simulink model "rlQubeServo"  (R2025a)
settings: Solver=ode23t  StartTime=0.0  StopTime=10.0  RelTol=1e-3  AbsTol=1e-3
values from neighbouring files (symbols this model uses):
  dphi0 = 0    [TrainAgentsToControlQuanserQUBEPendulumExample.m]    (also in training_1.mat)
  dtheta0 = 0    [TrainAgentsToControlQuanserQUBEPendulumExample.m]    (also in training_1.mat)
  dtheta_limit = 30    [TrainAgentsToControlQuanserQUBEPendulumExample.m]    (also in training_1.mat)
  phi0 = pi-pi/4+rand*pi/2    [TrainAgentsToControlQuanserQUBEPendulumExample.m]    (also in training_1.mat = 0)
  theta0 = -pi/4+rand*pi/2    [TrainAgentsToControlQuanserQUBEPendulumExample.m]    (also in training_1.mat = 0)
  theta_limit = 5*pi/8    (= 1.96349540849)    [TrainAgentsToControlQuanserQUBEPendulumExample.m]    (also in training_1.mat)
  Ts = 0.005    [TrainAgentsToControlQuanserQUBEPendulumExample.m]    (also in training_1.mat)
  volt_limit = 12    [TrainAgentsToControlQuanserQUBEPendulumExample.m]    (also in training_1.mat)
libraries: simulink x2, QuanserQube x1, rllib x1
settings Model: Creator=The MathWorks, Inc.  LastModifiedBy=The MathWorks, Inc.
settings SolverCC: AutoScaleAbsTol=off  MaxZcPerStep=1.0
settings DebuggingCC: UnconnectedInputMsg=warning  UnconnectedOutputMsg=warning  UnconnectedLineMsg=warning
settings ModelReferenceCC: EnableRefExpFcnMdlSchedulingChecks=on
settings RTWCC: GPUComputeCapability=3.5  DLArmComputeVersion=19.05
settings ExplorerConfigSet: InternalSimMechanicsExplorerSettings="<ExplorerConfiguration><canonicalview>default</canonicalview><AnimationSetting><BasePlaybackSpeed>1.0</BasePlaybackSpeed><PlaybackSpeedFactor>1.0</PlaybackSpeedFactor></AnimationSetting><TilePanel><TileInfo><Tiles Columns=\"1\" Count=\"1\" Rows=\"1\"><Column Weight=\"1\"/><Row Weight=\"1\"/><Tile Height=\"1\" Width=\"1\" X=\"0\" Y=\"0\"/></Tiles></TileInfo><SceneInfo><SceneViewer><BGColor><R>0.60000002384185791</R><G>0.60000002384185791</G><B>0.60000002384185791</B></BGColor><Camera><DoPerspective>on</DoPerspective><Position><X>0.334156231583514596</X><Y>0.107146061295956732</Y><Z>0.154419804164132285</Z></Position><Center><X>0.145480827141795971</X><Y>0.0537418892551446009</Y><Z>0.077934111254939889</Z></Center><Up><X>-0.332530024195597795</X><Y>-0.157027945704575345</Y><Z>0.929927958110882913</Z></Up><ViewLimDist>1</ViewLimDist><YLim>0.466307658154998583</YLim><XLim>0.535390274177961367</XLim></Camera></SceneViewer></SceneInfo></TilePanel><MechEditorPanel><Cameras><Camera><Id>Camera1</Id><Value><Name>Camera1</Name><NativeCamera><PositionKeyframeSet/><CenterKeyframeSet/><UpVectorKeyframeSet/></NativeCamera></Value></Camera></Cameras><GfxPanelCameraMap><MapElement CameraMLId=\"Camera1\" GfxPanelIndex=\"0\"/></GfxPanelCameraMap><VideoCreator><PlaybackSpeedRatio>1.0</PlaybackSpeedRatio><FrameRate>30</FrameRate><VideoFormat>Motion JPEG AVI</VideoFormat><FrameSize>auto</FrameSize></VideoCreator></MechEditorPanel></ExplorerConfiguration>"

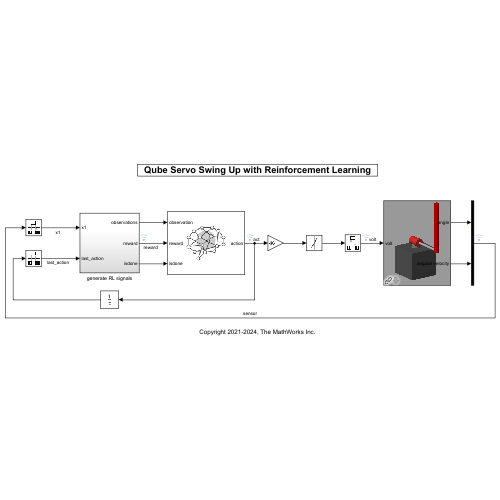
[thumbnail: Simulink's stored preview of the top-level diagram]
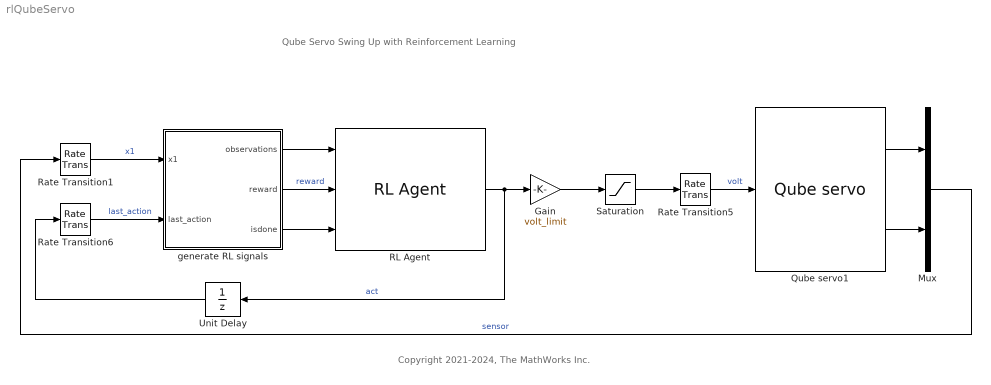
== system rlQubeServo ==
  note: Qube Servo Swing Up with Reinforcement Learning
  note: Copyright 2021-2024, The MathWorks Inc.
  Gain : Gain  Gain=volt_limit
  Mux : Mux  Inputs=2
  Qube servo1 : QuanserQube/Qube servo  a0=[theta0, phi0]  w0=[dtheta0,dphi0]  R_m=8.4  L_m=1.16e-3  mu_m=3e-6  K_b=0.042  n=1  rod_mass=0.095  rod_length=0.103  rod_rad=0.003  p_mass=0.024  p_length=0.129  p_rad=0.0045  D_r=0.001  D_p=5e-6  Choice_Stopper=On
  RL Agent : rllib/RL Agent  Agent=agent  ExternalActionAsInput=off  ProvideLastAction=off  ProvideCumRwd=off  TreatAsDirectFeedthrough=on  UseStrictObservationDataTypes=off
  Rate Transition1 : RateTransition  OutPortSampleTime=Ts
  Rate Transition5 : RateTransition
  Rate Transition6 : RateTransition  OutPortSampleTime=Ts
  Saturation : Saturate  UpperLimit=volt_limit  LowerLimit=-volt_limit
  Unit Delay : UnitDelay  SampleTime=-1  HasFrameUpgradeWarning=on
  generate RL signals : Subsystem
  wires:
  generate RL signals/3(isdone) -> RL Agent/3
  generate RL signals/2(reward) -> RL Agent/2  "reward"
  Qube servo1/1 -> Mux/1
  RL Agent/1 -> Gain/1, Unit Delay/1  "act"
  Qube servo1/2 -> Mux/2
  generate RL signals/1(observations) -> RL Agent/1
  Rate Transition1/1 -> generate RL signals/1(x1)  "x1"
  Unit Delay/1 -> Rate Transition6/1
  Mux/1 -> Rate Transition1/1  "sensor"
  Rate Transition6/1 -> generate RL signals/2(last_action)  "last_action"
  Saturation/1 -> Rate Transition5/1
  Rate Transition5/1 -> Qube servo1/1  "volt"
  Gain/1 -> Saturation/1

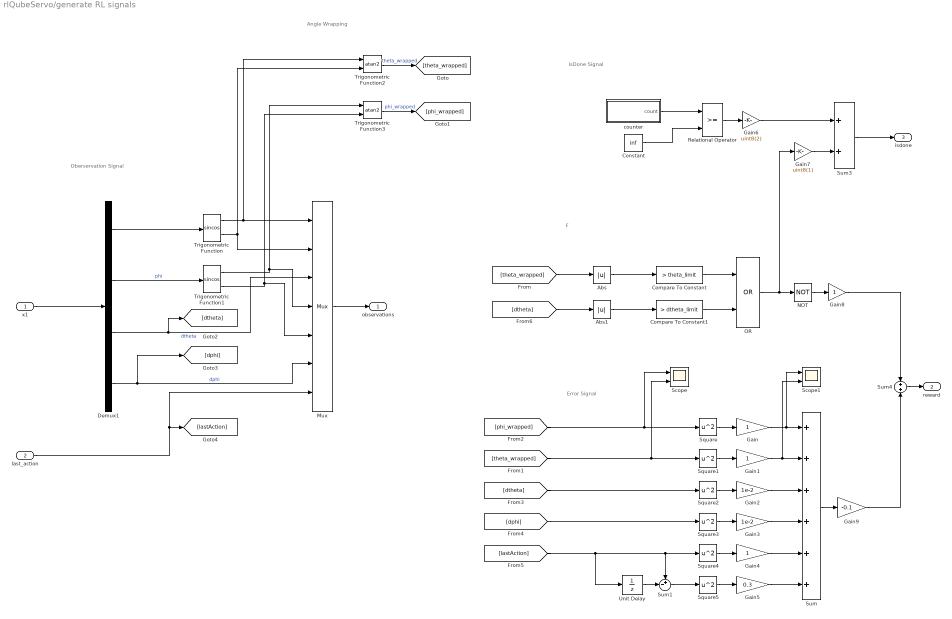
== system rlQubeServo/generate RL signals ==
  note: Oberservation Signal
  note: Error Signal
  note: isDone Signal
  note: Angle Wrapping
  note: F
  x1 : Inport  SampleTime=Ts
  last_action : Inport  Port=2
  Abs : Abs  SaturateOnIntegerOverflow=off
  Abs1 : Abs  SaturateOnIntegerOverflow=off
  Compare To Constant : simulink/Logic and Bit Operations/Compare To Constant  relop=>  const=theta_limit  OutDataTypeStr=boolean
  Compare To Constant1 : simulink/Logic and Bit Operations/Compare To Constant  relop=>  const=dtheta_limit  OutDataTypeStr=boolean
  Constant : Constant  Value=inf
  Demux1 : Demux
  Gain : Gain
  Gain1 : Gain
  Gain2 : Gain  Gain=1e-2
  Gain3 : Gain  Gain=1e-2
  Gain4 : Gain
  Gain5 : Gain  Gain=0.3
  Gain6 : Gain  Gain=uint8(2)  OutDataTypeStr=uint8
  Gain7 : Gain  Gain=uint8(1)  OutDataTypeStr=uint8
  Gain8 : Gain  OutDataTypeStr=double
  Gain9 : Gain  Gain=-0.1
  Mux : Mux  Inputs=7
  NOT : Logic  Operator=NOT  IconShape=distinctive  AllPortsSameDT=off  OutDataTypeStr=boolean
  OR : Logic  Operator=OR  IconShape=distinctive  AllPortsSameDT=off  OutDataTypeStr=boolean
  Relational Operator : RelationalOperator  OutDataTypeStr=boolean  RndMeth=Simplest  InputSameDT=off
  Scope : Scope  NumInputPorts=2
      settings: ActiveDisplayYMinimum=-0.2557  ActiveDisplayYMaximum=0.30688
  Scope1 : Scope  NumInputPorts=2
      settings: ActiveDisplayYMinimum=-3.92812  ActiveDisplayYMaximum=35.35621
  Square{,1..5} (6 alike) : Math  Operator=square
  Sum : Sum  Inputs=++++++
  Sum1 : Sum  Inputs=+-|
  Sum3 : Sum
  Sum4 : Sum
  Trigonometric Function : Trigonometry  Operator=sincos
  Trigonometric Function1 : Trigonometry  Operator=sincos
  Trigonometric Function2 : Trigonometry  Operator=atan2
  Trigonometric Function3 : Trigonometry  Operator=atan2
  Unit Delay : UnitDelay  SampleTime=-1  HasFrameUpgradeWarning=on
  counter : Subsystem
  observations : Outport
  reward : Outport  Port=2
  isdone : Outport  Port=3
  wires:
  Square3/1 -> Gain3/1
  Trigonometric Function1/1 -> Mux/4, Trigonometric Function3/1
  Compare To Constant/1 -> OR/1
  Square1/1 -> Gain1/1
  Gain9/1 -> Sum4/2
  Unit Delay/1 -> Sum1/2
  Trigonometric Function2/1 -> [theta_wrapped]  "theta_wrapped"
  Gain4/1 -> Sum/5
  Mux/1 -> observations/1
  Gain5/1 -> Sum/6
  Trigonometric Function1/2 -> Mux/5, Trigonometric Function3/2
  OR/1 -> Gain7/1, NOT/1
  Compare To Constant1/1 -> OR/2
  Square5/1 -> Gain5/1
  Gain8/1 -> Sum4/1
  Square/1 -> Gain/1
  Demux1/4 -> [dphi], Mux/6  "dphi"
  NOT/1 -> Gain8/1
  Square4/1 -> Gain4/1
  Gain1/1 -> Scope1/2, Sum/2
  Sum4/1 -> reward/1
  counter/1(count) -> Relational Operator/1
  Trigonometric Function/2 -> Trigonometric Function2/2, Mux/2
  x1/1 -> Demux1/1
  Relational Operator/1 -> Gain6/1
  Constant/1 -> Relational Operator/2
  Sum3/1 -> isdone/1
  Trigonometric Function/1 -> Mux/1, Trigonometric Function2/1
  Abs1/1 -> Compare To Constant1/1
  Sum/1 -> Gain9/1
  Square2/1 -> Gain2/1
  Sum1/1 -> Square5/1
  Abs/1 -> Compare To Constant/1
  Demux1/3 -> [dtheta], Mux/3  "dtheta"
  Gain2/1 -> Sum/3
  Gain3/1 -> Sum/4
  Gain/1 -> Scope1/1, Sum/1
  Demux1/1 -> Trigonometric Function/1
  Demux1/2 -> Trigonometric Function1/1  "phi"
  [theta_wrapped] -> Abs/1
  last_action/1 -> Mux/7, [lastAction]
  [theta_wrapped] -> Scope/2, Square1/1
  Trigonometric Function3/1 -> [phi_wrapped]  "phi_wrapped"
  [phi_wrapped] -> Scope/1, Square/1
  [dtheta] -> Square2/1
  [dphi] -> Square3/1
  [lastAction] -> Sum1/1, Square4/1, Unit Delay/1
  [dtheta] -> Abs1/1
  Gain6/1 -> Sum3/1
  Gain7/1 -> Sum3/2

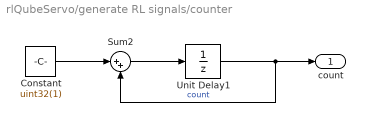
== system rlQubeServo/generate RL signals/counter ==
  Constant : Constant  Value=uint32(1)
  Sum2 : Sum  Inputs=|++
  Unit Delay1 : UnitDelay  SampleTime=Ts  HasFrameUpgradeWarning=on
  count : Outport  OutDataTypeStr=uint32
  wires:
  Sum2/1 -> Unit Delay1/1
  Unit Delay1/1 -> count/1, Sum2/2  "count"
  Constant/1 -> Sum2/1
